simulink model "AMCLIB_SpeedLoop_BAM_F32"  (Simulink 8.3)
settings: Solver=ode45  StartTime=0.0  StopTime=10.0  RelTol=1e-3
undefined symbols (not defined in the file): f32IntegGainQ, f32PropGainQ, f32RampDown, f32RampUp, s16IntegGainShiftQ, s16PropGainShiftQ, u16NSamplesW
settings Model: Creator=B37097  LastModifiedBy=B37097
settings DataIOCC: SignalLoggingSaveFormat=Dataset
settings DebuggingCC: UnderspecifiedInitializationDetection=Simplified  StateNameClashWarn=none
settings GRTTargetCC: CombineOutputUpdateFcns=on  GRTInterface=off

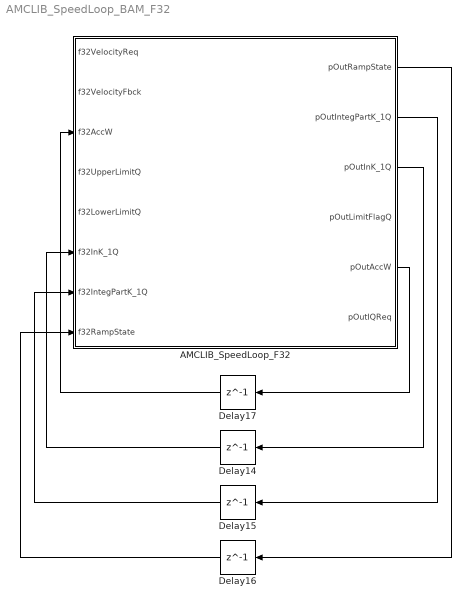
== system AMCLIB_SpeedLoop_BAM_F32 ==
  AMCLIB_SpeedLoop_F32 : Subsystem  mask(AMCLIB_SpeedLoop_F32){u16NSamplesW=u16NSamplesW, f32PropGainQ=f32PropGainQ, s16PropGainShiftQ=s16PropGainShiftQ, f32IntegGainQ=f32IntegGainQ, s16IntegGainShiftQ=s16IntegGainShiftQ, f32RampUp=f32RampUp, f32RampDown=f32RampDown}
      mask help: Bit accurate model of the speed loop algorithm with field weakening capability in 32-bit fixed-point implementation.
      mask init:
      | pos = get_param(gcb, 'Position');width = pos(3) - pos(1); height = pos(4) - pos(2);tX=width/2;tY=height*0.9;
      mask Display: color('black');port_label('input',1,'f32VelocityReq');port_label('input',2,'f32VelocityFbck');port_label('input',3,'f32AccW');port_label('input',4,'f32UpperLimitQ');port_label('input',5,'f32LowerLimitQ');port_label('input',6,'f32InK_1Q');port_label('input',7,'f32IntegPartK_1Q');port_label('input',8,'f32RampState');port_label('output',1,'pOutRampState');port_label('output',2,'pOutIntegPartK_1Q');port_label('output',3,'pOutInK_1Q');port_label('output',4,'pOutLimitFlagQ');port_label('output',5,'pOutAccW');port_label('output',6,'pOutIQReq');color('black');disp('AMCLIB_SpeedLoop_F32');color('blue');text(tX,tY, 'BAM', 'horizontalAlignment', 'center');
  Delay{14..17} (4 alike) : Delay  DelayLength=1  InitialCondition=0
  wires:
  AMCLIB_SpeedLoop_F32/5(pOutAccW) -> Delay17/1
  AMCLIB_SpeedLoop_F32/3(pOutInK_1Q) -> Delay14/1
  AMCLIB_SpeedLoop_F32/2(pOutIntegPartK_1Q) -> Delay15/1
  AMCLIB_SpeedLoop_F32/1(pOutRampState) -> Delay16/1
  Delay17/1 -> AMCLIB_SpeedLoop_F32/3(f32AccW)
  Delay14/1 -> AMCLIB_SpeedLoop_F32/6(f32InK_1Q)
  Delay15/1 -> AMCLIB_SpeedLoop_F32/7(f32IntegPartK_1Q)
  Delay16/1 -> AMCLIB_SpeedLoop_F32/8(f32RampState)

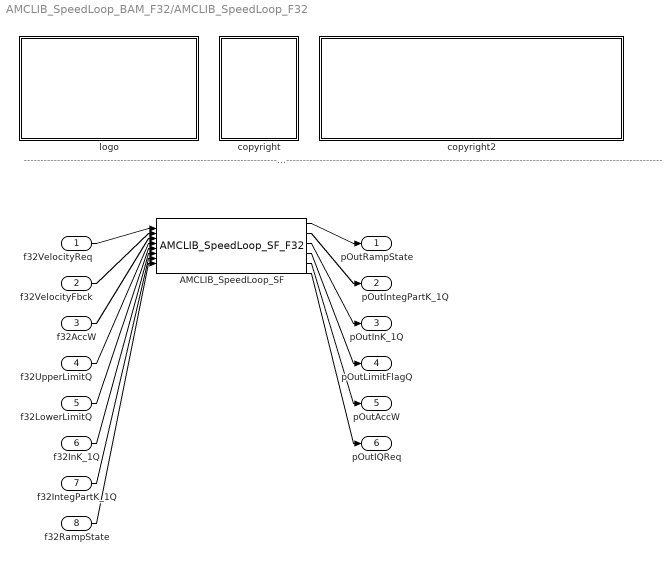
== system AMCLIB_SpeedLoop_BAM_F32/AMCLIB_SpeedLoop_F32 ==
  note: ---------------------------------------------------------------------------------------------------------------------------------------------------------------------------------------------------
  f32VelocityReq : Inport
  f32VelocityFbck : Inport  Port=2
  f32AccW : Inport  Port=3
  f32UpperLimitQ : Inport  Port=4
  f32LowerLimitQ : Inport  Port=5
  f32InK_1Q : Inport  Port=6
  f32IntegPartK_1Q : Inport  Port=7
  f32RampState : Inport  Port=8
  AMCLIB_SpeedLoop_SF : S-Function  FunctionName=AMCLIB_SpeedLoop_SF_F32  Parameters=u16NSamplesW,f32PropGainQ,s16PropGainShiftQ,f32IntegGainQ,s16IntegGainShiftQ,f32RampUp,f32RampDown  EnableBusSupport=off
  copyright : Subsystem
      mask Display: text(10,90,'FILE:');text(10,75,'DESRIPTION:');text(10,60,'COPYRIGHT:');text(10,45,'VERSION:');text(10,30,'DATE:')
  copyright2 : Subsystem
      mask Display: text(10,90,'AMCLIB_SpeedLoop_BAM_F32.mdl');text(10,75,'Speed Loop with Field Weakening.');text(10,60,'NXP');text(10,45,'1.0');text(10,30,'28-Aug-2017');
  logo : Subsystem
      mask Display: image(imread('logo.jpg'))
  pOutRampState : Outport
  pOutIntegPartK_1Q : Outport  Port=2
  pOutInK_1Q : Outport  Port=3
  pOutLimitFlagQ : Outport  Port=4
  pOutAccW : Outport  Port=5
  pOutIQReq : Outport  Port=6
  wires:
  f32VelocityReq/1 -> AMCLIB_SpeedLoop_SF/1
  f32VelocityFbck/1 -> AMCLIB_SpeedLoop_SF/2
  f32AccW/1 -> AMCLIB_SpeedLoop_SF/3
  f32UpperLimitQ/1 -> AMCLIB_SpeedLoop_SF/4
  f32LowerLimitQ/1 -> AMCLIB_SpeedLoop_SF/5
  f32InK_1Q/1 -> AMCLIB_SpeedLoop_SF/6
  f32IntegPartK_1Q/1 -> AMCLIB_SpeedLoop_SF/7
  f32RampState/1 -> AMCLIB_SpeedLoop_SF/8
  AMCLIB_SpeedLoop_SF/1 -> pOutRampState/1
  AMCLIB_SpeedLoop_SF/2 -> pOutIntegPartK_1Q/1
  AMCLIB_SpeedLoop_SF/3 -> pOutInK_1Q/1
  AMCLIB_SpeedLoop_SF/4 -> pOutLimitFlagQ/1
  AMCLIB_SpeedLoop_SF/5 -> pOutAccW/1
  AMCLIB_SpeedLoop_SF/6 -> pOutIQReq/1

== system AMCLIB_SpeedLoop_BAM_F32/AMCLIB_SpeedLoop_F32/copyright ==

== system AMCLIB_SpeedLoop_BAM_F32/AMCLIB_SpeedLoop_F32/copyright2 ==

== system AMCLIB_SpeedLoop_BAM_F32/AMCLIB_SpeedLoop_F32/logo ==
